simulink model "s433b"  (Simulink 5.1)
settings: Solver=ode45  StartTime=0.0  StopTime=100.0  RelTol=1e-3
settings Model: LastModifiedBy=user_father  BooleanDataType=on  ProdHWDeviceType=Microprocessor

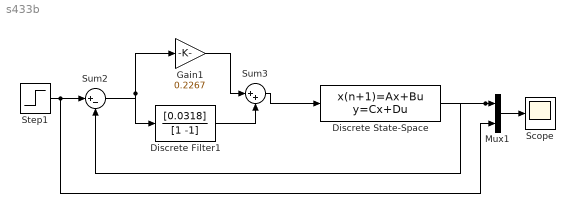
== system s433b ==
  Discrete Filter1 : DiscreteFilter  Numerator=[0.0318]  Denominator=[1 -1]
  Discrete State-Space : DiscreteStateSpace  A=[0.368 0;0.632 1]  B=[0.632;0.368]  C=[0 1]  D=0
  Gain1 : Gain  Gain=0.2267  SaturateOnIntegerOverflow=on
  Mux1 : Mux  Inputs=2
  Scope : Scope
  Step1 : Step  Time=0  SampleTime=0
  Sum2 : Sum  Inputs=|+-  SaturateOnIntegerOverflow=on
  Sum3 : Sum  Inputs=|++  SaturateOnIntegerOverflow=on
  wires:
  Step1/1 -> Sum2/1, Mux1/2
  Sum2/1 -> Gain1/1, Discrete Filter1/1
  Sum3/1 -> Discrete State-Space/1
  Discrete Filter1/1 -> Sum3/2
  Gain1/1 -> Sum3/1
  Mux1/1 -> Scope/1
  Discrete State-Space/1 -> Sum2/2, Mux1/1
